simulink model "ahu_grejac_model"  (R2021a)
settings: Solver=VariableStepAuto  StartTime=0.0  StopTime=10000  RelTol=1e-3
model workspace (MATLAB code in the model file):
  | % Paramtri za model zone
  | C_z = 47.1;                % kJ/ C
  | C_pa = 1.005;            % kJ/(kg C)
  | C_w1 = 70;               % kJ / C
  | C_w2 = 60;               % kJ / C
  | C_R = 80;                % kJ / C
  | f_sa = 0.192;            % m^3 / s
  | Ro_a = 1.25;             % kg / m^3
  | U_w1 = 2;                % W / (m^2 C)
  | U_w2 = 2;                % W / (m^2 C)
  | U_R = 1;                 % W / (m^2 C)
  | A_R = 9;                 % m^2
  | A_w1 = 9;                % m^2
  | A_w2 = 12;               % m^2
  | 
  | % Parametri potrebni za model grejaca
  | T_wo = 10;
  | T_o = 5;
  | %Twi i Tm se racunaju
  | C_ah = 4.5;              % kJ/C
  | C_pw = 4.1868;           % kJ/(kg C)
  | f_sw = 0.0000802;          % m^3 / s
  | Ro_w = 998;              % kg / m^3
  | UA_a = 0.04;             % kJ / s C
  | T_zeljeno = 22;
  | m_r = 0.12;              % kg / s
  | m_o = 0.12;              % kg / s
libraries: slpidlib x1
settings Model: OrderedModelArguments=off

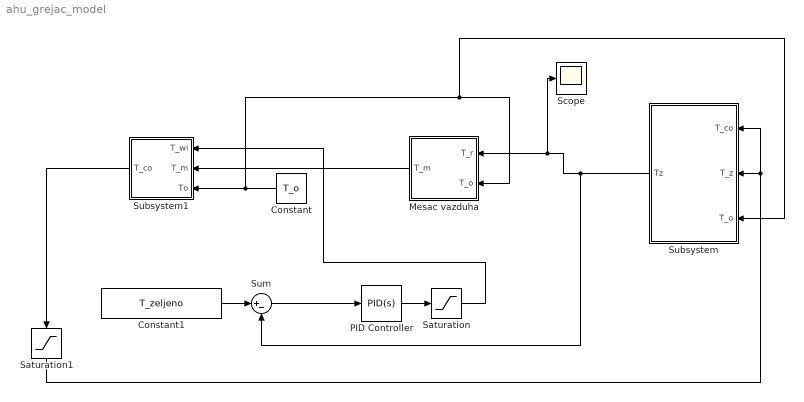
== system ahu_grejac_model ==
  Constant : Constant  Value=T_o
  Constant1 : Constant  Value=T_zeljeno
  Mesac vazduha : Subsystem
  PID Controller : slpidlib/PID Controller  Controller=PID  Form=Parallel  TimeDomain=Continuous-time  UseExternalTs=off  SampleTime=-1  IntegratorMethod=Forward Euler  FilterMethod=Forward Euler  ControllerParametersSource=internal  P=5  I=1  D=0  UseFilter=on  N=100  TunerSelectOption=Transfer Function Based (PID Tuner App)  InitialConditionSource=internal  InitialConditionForIntegrator=0  InitialConditionForFilter=0  DifferentiatorICPrevScaledInput=0  ExternalReset=none  TrackingMode=off  Kt=1  LimitOutput=off  SatLimitsSource=internal  UpperSaturationLimit=inf  LowerSaturationLimit=-inf  LinearizeAsGain=on  AntiWindupMode=none  Kb=1  POutMin=[]  POutMax=[]  IOutMin=[]  IOutMax=[]  DOutMin=[]  DOutMax=[]  NOutMin=[]  NOutMax=[]  SumOutMin=[]  SumOutMax=[]  SaturationOutMin=[]  SaturationOutMax=[]  PParamMin=[]  PParamMax=[]  IParamMin=[]  IParamMax=[]  DParamMin=[]  DParamMax=[]  NParamMin=[]  NParamMax=[]  KbParamMin=[]  KbParamMax=[]  KtParamMin=[]  KtParamMax=[]  KbOutMin=[]  KbOutMax=[]  KtOutMin=[]  KtOutMax=[]  IntegratorOutMin=[]  IntegratorOutMax=[]  FilterOutMin=[]  FilterOutMax=[]  SumI1OutMin=[]  SumI1OutMax=[]  SumI2OutMin=[]  SumI2OutMax=[]  SumI3OutMin=[]  SumI3OutMax=[]  SumI4OutMin=[]  SumI4OutMax=[]  SumDOutMin=[]  SumDOutMax=[]  DifferentiatorOutMin=[]  DifferentiatorOutMax=[]  FilterDiffOutCoefMin=[]  FilterDiffOutCoefMax=[]  ReciprocalOutMin=[]  ReciprocalOutMax=[]  SumDenOutMin=[]  SumDenOutMax=[]  SumNumOutMin=[]  SumNumOutMax=[]  DivideOutMin=[]  DivideOutMax=[]  UdiffTsProdOutMin=[]  UdiffTsProdOutMax=[]  NTsProdOutMin=[]  NTsProdOutMax=[]  UintegralTsProdOutMin=[]  UintegralTsProdOutMax=[]  UngainTsProdOutMin=[]  UngainTsProdOutMax=[]  IntegratorContinuousStateAttributes=''  IntegratorStateMustResolveToSignalObject=off  IntegratorRTWStateStorageClass=Auto  FilterContinuousStateAttributes=''  FilterStateMustResolveToSignalObject=off  FilterRTWStateStorageClass=Auto  ParallelPVariant=InternalParameters  IdealPVariant=Disabled  IVariant=InternalParameters  DVariant=InternalParameters  IntegratorVariant=Continuous  SatVariant=Disabled  AWVariant=Passthrough  PCopyVariant=Disabled  TRVariant=Disabled  FdbkBlocksVariant=Forward  IdealPFdbkVariant=Disabled  SatFdbkVariant=Disabled  DerivativeFilterVariant=ContFilter  NVariant=InternalParameters  NCopyVariant=Disabled  FilterICVariant=InternalICsFilter  IntegratorICVariant=InternalICs  ExternalResetVariant=Disabled  TRSumVariant=Passthrough  SumFdbkVariant=Disabled  SumVariant=Sum_PID  TsampFilterVariant=InternalTs  TsampNgainVariant=Passthrough  TsampIntegralVariant=Passthrough  ExternalSaturationOutDataTypeStr=Inherit: Same as second input
  Saturation : Saturate  UpperLimit=50  LowerLimit=0
  Saturation1 : Saturate  UpperLimit=50  LowerLimit=0
  Scope : Scope
  Subsystem : Subsystem
  Subsystem1 : Subsystem
  Sum : Sum  Inputs=|+-
  wires:
  Constant1/1 -> Sum/1
  Sum/1 -> PID Controller/1
  PID Controller/1 -> Saturation/1
  Saturation/1 -> Subsystem1/1(T_wi)
  Subsystem1/1(T_co) -> Saturation1/1
  Mesac vazduha/1(T_m) -> Subsystem1/2(T_m)
  Subsystem/1(Tz) -> Sum/2, Scope/1, Mesac vazduha/1(T_r)
  Constant/1 -> Subsystem/3(T_o), Mesac vazduha/2(T_o), Subsystem1/3(To)
  Saturation1/1 -> Subsystem/2(T_z), Subsystem/1(T_co)

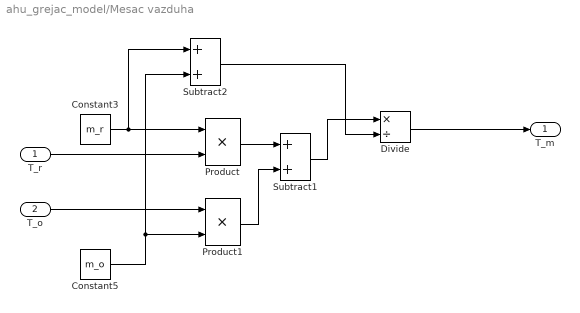
== system ahu_grejac_model/Mesac vazduha ==
  T_r : Inport
  T_o : Inport  Port=2
  Constant3 : Constant  Value=m_r
  Constant5 : Constant  Value=m_o
  Divide : Product  Inputs=*/
  Product : Product
  Product1 : Product
  Subtract1 : Sum
  Subtract2 : Sum
  T_m : Outport
  wires:
  Product1/1 -> Subtract1/2
  Constant3/1 -> Product/1, Subtract2/1
  Constant5/1 -> Product1/2, Subtract2/2
  Divide/1 -> T_m/1
  Subtract1/1 -> Divide/1
  T_r/1 -> Product/2
  Subtract2/1 -> Divide/2
  Product/1 -> Subtract1/1
  T_o/1 -> Product1/1

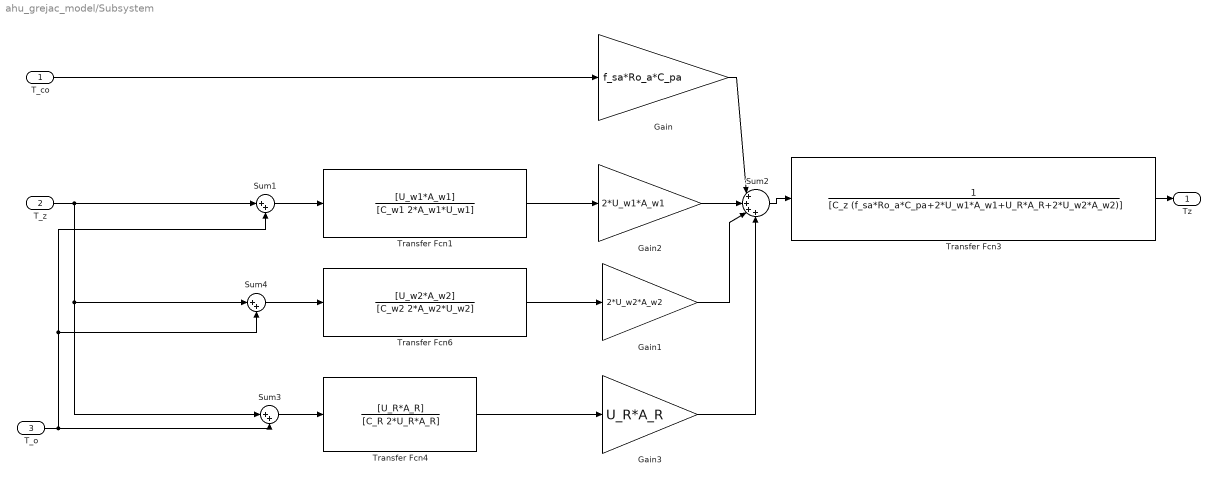
== system ahu_grejac_model/Subsystem ==
  T_co : Inport
  T_z : Inport  Port=2
  T_o : Inport  Port=3
  Gain : Gain  Gain=f_sa*Ro_a*C_pa
  Gain1 : Gain  Gain=2*U_w2*A_w2
  Gain2 : Gain  Gain=2*U_w1*A_w1
  Gain3 : Gain  Gain=U_R*A_R
  Sum1 : Sum  Inputs=|++
  Sum2 : Sum  Inputs=|++++
  Sum3 : Sum  Inputs=|++
  Sum4 : Sum  Inputs=|++
  Transfer Fcn1 : TransferFcn  Numerator=[U_w1*A_w1]  Denominator=[C_w1 2*A_w1*U_w1]
  Transfer Fcn3 : TransferFcn  Denominator=[C_z (f_sa*Ro_a*C_pa+2*U_w1*A_w1+U_R*A_R+2*U_w2*A_w2)]
  Transfer Fcn4 : TransferFcn  Numerator=[U_R*A_R]  Denominator=[C_R 2*U_R*A_R]
  Transfer Fcn6 : TransferFcn  Numerator=[U_w2*A_w2]  Denominator=[C_w2 2*A_w2*U_w2]
  Tz : Outport
  wires:
  Gain/1 -> Sum2/1
  Gain1/1 -> Sum2/3
  Transfer Fcn3/1 -> Tz/1
  Gain2/1 -> Sum2/2
  Sum2/1 -> Transfer Fcn3/1
  Transfer Fcn4/1 -> Gain3/1
  Sum3/1 -> Transfer Fcn4/1
  Sum1/1 -> Transfer Fcn1/1
  Gain3/1 -> Sum2/4
  Transfer Fcn6/1 -> Gain1/1
  T_o/1 -> Sum3/2, Sum1/2, Sum4/2
  Transfer Fcn1/1 -> Gain2/1
  Sum4/1 -> Transfer Fcn6/1
  T_co/1 -> Gain/1
  T_z/1 -> Sum3/1, Sum4/1, Sum1/1

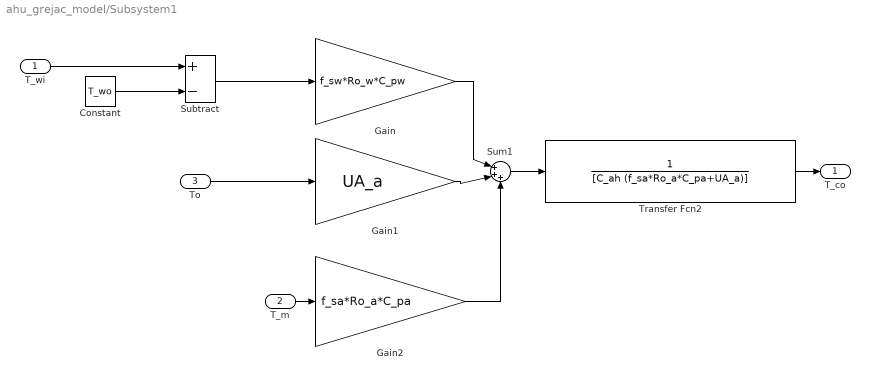
== system ahu_grejac_model/Subsystem1 ==
  T_wi : Inport
  T_m : Inport  Port=2
  To : Inport  Port=3
  Constant : Constant  Value=T_wo
  Gain : Gain  Gain=f_sw*Ro_w*C_pw
  Gain1 : Gain  Gain=UA_a
  Gain2 : Gain  Gain=f_sa*Ro_a*C_pa
  Subtract : Sum  Inputs=+-
  Sum1 : Sum  Inputs=|+++
  Transfer Fcn2 : TransferFcn  Denominator=[C_ah (f_sa*Ro_a*C_pa+UA_a)]
  T_co : Outport
  wires:
  Gain2/1 -> Sum1/3
  To/1 -> Gain1/1
  T_wi/1 -> Subtract/1
  Gain/1 -> Sum1/1
  Subtract/1 -> Gain/1
  T_m/1 -> Gain2/1
  Constant/1 -> Subtract/2
  Gain1/1 -> Sum1/2
  Sum1/1 -> Transfer Fcn2/1
  Transfer Fcn2/1 -> T_co/1
